simulink model "SWC_HALOUT_type_backup"  (R2021b)
settings: Solver=FixedStepDiscrete  StartTime=0.0  StopTime=10.0  FixedStep=0.001  RelTol=1e-3
undefined symbols (not defined in the file or in its folder): DIDLen_APPPedalZP, DIDLen_APSFunConfig, DIDLen_AutoLock, DIDLen_AutoWipHSpdEN, DIDLen_DKCKey, DIDLen_DRLDis, DIDLen_DynoMode, DIDLen_FMHTimer, DIDLen_LFLowPresThre, DIDLen_LFSensorID, DIDLen_LRLowPresThre, DIDLen_LRSensorID, DIDLen_NVMPedalZP, DIDLen_RFLowPresThre, DIDLen_RFSensorID, DIDLen_RRLowPresThre, DIDLen_RRSensorID, DIDLen_SensorMode, DIDLen_TireSize, DIDLen_TPMSLearnSta, DIDLen_TurnLampFLThreCurr, DIDLen_TurnLampFRThreCurr, DIDLen_TurnLampRLThreCurr, DIDLen_TurnLampRRThreCurr, DIDLen_USSConfig, DIDLen_WhlPres, DIDLen_WhlSensorBattSta, DIDLen_WhlTmp, DIDLen_WipRLSCmdCutFilter, DIDLen_WipRLSCmdHoldFilter, DIDLen_XWDMode, DIDNum_APPPedalZP, DIDNum_APSFunConfig, DIDNum_AutoLock, DIDNum_AutoWipHSpdEN, DIDNum_DKCKey, DIDNum_DRLDis, DIDNum_DynoMode, DIDNum_FMHTimer, DIDNum_LFLowPresThre, DIDNum_LFSensorID, DIDNum_LRLowPresThre, DIDNum_LRSensorID, DIDNum_NVMPedalZP, DIDNum_RFLowPresThre, DIDNum_RFSensorID, DIDNum_RRLowPresThre, DIDNum_RRSensorID, DIDNum_SensorMode, DIDNum_TireSize, DIDNum_TPMSLearnSta, DIDNum_TurnLampFLThreCurr, DIDNum_TurnLampFRThreCurr, DIDNum_TurnLampRLThreCurr, DIDNum_TurnLampRRThreCurr, DIDNum_USSConfig, DIDNum_WhlPres, DIDNum_WhlSensorBattSta, DIDNum_WhlTmp, DIDNum_WipRLSCmdCutFilter ... (+278)
libraries: FVT_lib x133, simulink x108, hdlsllib x6, hcu_lib x5, halout x1
(part 2 of 7)

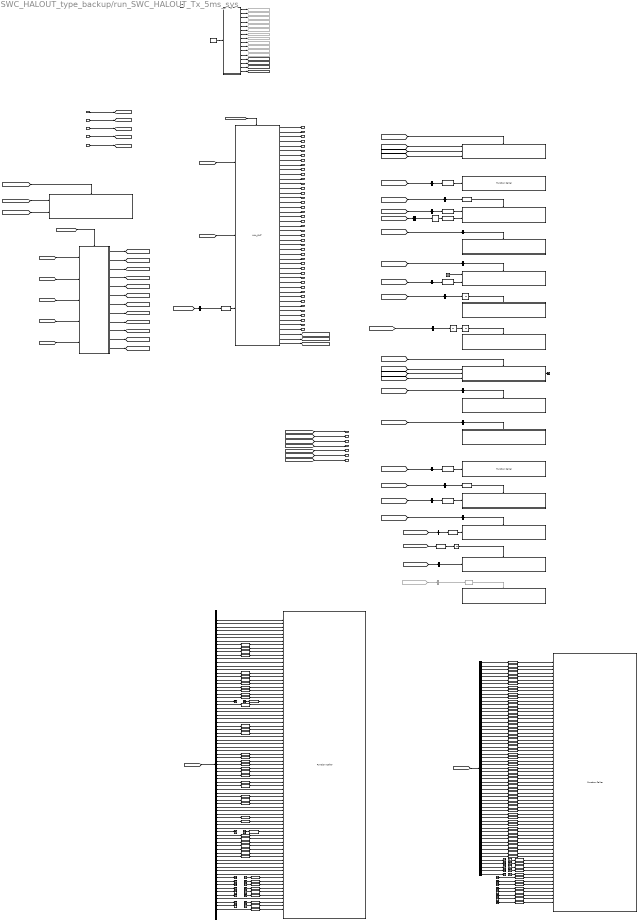
== system SWC_HALOUT_type_backup/run_SWC_HALOUT_Tx_5ms_sys ==
  R_BSCP_outputs_BSCP_outputs_read : Inport
  R_BOUTP_outputs_BOUTP_outputs_read : Inport  Port=2
  R_BHAL_SYS_outputs_BHAL_SYS_outputs_read : Inport  Port=3
  R_BHAL_DID_outputs_BHAL_DID_outputs_read : Inport  Port=4
  R_NVMReadCDD_u8Array1024_NVMReadData_read : Inport  Port=5
  function : TriggerPort  TriggerType=function-call  VariantControl=(inherit)  SampleTimeType=periodic  SampleTime=-1
  Bus Selector15 : BusSelector  OutputSignals=VHAL_AcoreReadyToSlp_flg
  Bus Selector3 : BusSelector  OutputSignals=VOUTP_PowerSta_enum,VOUTP_BrkPedalPos_pct,VOUTP_ActAPSPosn_pct,VOUTP_LFRawWhlSpeed_kph,VOUTP_RFRawWhlSpeed_kph,VOUTP_LRRawWhlSpeed_kph,VOUTP_RRRawWhlSpeed_kph,VOUTP_LFRawWhlSpeedV_flg,VOUTP_RFRawWhlSpeedV_flg,VOUTP_LRRawWhlSpeedV_flg,VOUTP_RRRawWhlSpeedV_flg,VOUTP_LFWhlRotDir_enum,VOUTP_RFWhlRotDir_enum,VOUTP_LRWhlRotDir_enum,VOUTP_RRWhlRotDir_enum,VOUTP_LFPulseCountV_flg,VOUTP_RFPulseCountV_flg,VOUTP_LRPulseCountV_flg,VOUTP_RRPulseCountV_flg,VOUTP_LFPulseCount_enum,VOUTP_RFPulseCount_enum,VOUTP_LRPulseCount_enum,VOUTP_RRPulseCount_enum,VOUTP_VehSpeed_kph,VOUTP_APSCtrlAvail_flg,VOUTP_ShifterHandleCmd_enum,VOUTP_DriIntend_enum,VOUTP_EPSAOIControl_enum,VOUTP_SASAngle_Deg,VOUTP_SASSpeed_degps,VOUTP_SASSpeedValid_flg,VOUTP_SASCAL_flg,VOUTP_SASV_flg,VOUTP_GRADE_Deg,VOUTP_YawRate_degps,VOUTP_LatAccel_Gps,VOUTP_LongAccel_Gps,VOUTP_MCPressure_bar,VOUTP_YawRateV_flg,VOUTP_LatAccelV_flg,VOUTP_LongAccelV_flg,VOUTP_MCPressureV_bar,VOUTP_BrkSwSta_flg,VOUTP_BrkSwV_flg,VOUTP_ESCStandstill_flg,VOUTP_ESCAPSSta_enum,VOUTP_EPBExtReleaseAvail_flg,VOUTP_EPBExtApplyAvail_flg,VOUTP_EPBErrSta_enum,VOUTP_EPBSta_enum,VOUTP_AllDoorSW_flg,VOUTP_HoodSW_flg,VOUTP_TailgateSW_flg,VOUTP_AVMparkingcancel_enum,VOUTP_AVMparkingexcute_enum,VOUTP_AVMParkingmode_enum,VOUTP_AVMErrSTA_flg,VOUTP_IVIStatus_flg,VOUTP_CAASSw_enum,VOUTP_IVIScreen_enum,VOUTP_VehSpeedTimeOut_flg,VOUTP_ABSActive_flg,VOUTP_TCSActive_flg,VOUTP_DriverSeatBeltCmd_flg,VOUTP_DrDoorSW_flg,VOUTP_PsDoorSW_flg,VOUTP_RLDoorSW_flg,VOUTP_RRDoorSW_flg,VOUTP_RFPressIndi_enum,VOUTP_LFPressIndi_enum,VOUTP_RRPressIndi_enum,VOUTP_LRPressIndi_enum,VOUTP_sigAmbAirT_C,VOUTP_FSOffSw_enum,VOUTP_FSOffSwTimeOut_flg,VOUTP_VehSpeed_kph,VOUTP_VehSpeed_kph,VOUTP_VehSpeed_kph,VOUTP_VehSpeed_kph,VOUTP_DrSeatSta_enum,VOUTP_VehSpeed_kph,VOUTP_VehSpeed_kph,VOUTP_IVIUserTakeOverAPSSta_flg
  Bus Selector4 : BusSelector  OutputSignals=VOUTP_BrkPedalPosTimeOut_flg,VOUTP_LFRawWhlSpeedTimeOut_flg,VOUTP_RFRawWhlSpeedTimeOut_flg,VOUTP_LRRawWhlSpeedTimeOut_flg,VOUTP_RRRawWhlSpeedTimeOut_flg,VOUTP_LFRawWhlSpeedVTimeOut_flg,VOUTP_RFRawWhlSpeedVTimeOut_flg,VOUTP_LRRawWhlSpeedVTimeOut_flg,VOUTP_RRRawWhlSpeedVTimeOut_flg,VOUTP_LFWhlRotDirTimeOut_flg,VOUTP_RFWhlRotDirTimeOut_flg,VOUTP_LRWhlRotDirTimeOut_flg,VOUTP_RRWhlRotDirTimeOut_flg,VOUTP_LFPulseCountVTimeOut_flg,VOUTP_RFPulseCountVTimeOut_flg,VOUTP_LRPulseCountVTimeOut_flg,VOUTP_RRPulseCountVTimeOut_flg,VOUTP_LFPulseCountTimeOut_flg,VOUTP_RFPulseCountTimeOut_flg,VOUTP_LRPulseCountTimeOut_flg,VOUTP_RRPulseCountTimeOut_flg,VOUTP_ShifterHandleCmdTimeOut_flg,VOUTP_DriIntendTimeOut_flg,VOUTP_EPSAOIControlTimeOut_flg,VOUTP_SASAngleTimeOut_flg,VOUTP_SASSpeedTimeOut_flg,VOUTP_SASSpeedValidTimeOut_flg,VOUTP_SASCALTimeOut_flg,VOUTP_SASVTimeOut_flg,VOUTP_GRADETimeOut_flg,VOUTP_YawRateTimeOut_flg,VOUTP_LatAccelTimeOut_flg,VOUTP_LongAccelTimeOut_flg,VOUTP_MCPressureTimeOut_flg,VOUTP_YawRateVTimeOut_flg,VOUTP_LatAccelVTimeOut_flg,VOUTP_LongAccelVTimeOut_flg,VOUTP_MCPressureVTimeOut_flg,VOUTP_BrkSwStaTimeOut_flg,VOUTP_BrkSwVTimeOut_flg,VOUTP_ESCStandstillTimeOut_flg,VOUTP_ESCAPSStaTimeOut_flg,VOUTP_EPBExtReleaseAvailTimeOut_flg,VOUTP_EPBExtApplyAvailTimeOut_flg,VOUTP_EPBErrStaTimeOut_flg,VOUTP_EPBStaTimeOut_flg,VOUTP_AVMparkingcancelTimeOut_flg,VOUTP_AVMparkingexcuteTimeOut_flg,VOUTP_AVMParkingmodeTimeOut_flg,VOUTP_AVMErrSTATimeOut_flg,VOUTP_IVIStatusTimeOut_flg,VOUTP_CAASSwTimeOut_flg,VOUTP_IVIScreenTimeOut_flg,VOUTP_ABSActiveTimeOut_flg,VOUTP_TCSActiveTimeOut_flg,VOUTP_DriverSeatBeltCmdTimeOut_flg,VOUTP_RFPressIndi_enum,VOUTP_LFPressIndi_enum,VOUTP_RRPressIndi_enum,VOUTP_LRPressIndi_enum,VOUTP_sigAmbAirT_C
  Bus Selector6 : BusSelector  OutputSignals=VHAL_TPMSSensorIDRegResults_raw8
  Bus Selector8 : BusSelector  Commented=on  OutputSignals=VOUTP_ResetPedalZeroPosStart_flg
  Bus Selector9 : BusSelector  OutputSignals=VHAL_DIDSetNVMPedalZP_raw8
  Constant5 : Constant  Value=FALSE
  DIDSet_Subsystem : Subsystem
  Data Type Conversion{,1..2,4..5,7..13,17..19,21..107,109..125} (119 alike) : DataTypeConversion  OutDataTypeStr=uint8
  Data Type Conversion108 : DataTypeConversion  OutDataTypeStr=boolean
  Data Type Conversion{14..16,20} (4 alike) : DataTypeConversion  OutDataTypeStr=int16
  Data Type Conversion3 : DataTypeConversion  OutDataTypeStr=uint32
  Data Type Conversion6 : DataTypeConversion  OutDataTypeStr=single
  Detect Increase1 : simulink/Logic and Bit Operations/Detect Increase  Commented=on  vinit=0.0  OutDataTypeStr=boolean
  From139 : From  Commented=on  GotoTag=BOUTP_outputs
  Goto100 : Goto  Commented=on  GotoTag=trig_Read_NVM_00
  Goto102 : Goto  Commented=on  GotoTag=trig_ReadIMUOffset_00
  Goto106 : Goto  Commented=on  GotoTag=trig_GetNMID
  Goto119 : Goto  Commented=on  GotoTag=trig_HAL_DKC_10_3
  Goto90 : Goto  Commented=on  GotoTag=trig_GetDID
  Goto91 : Goto  Commented=on  GotoTag=trig_WDG
  Goto92 : Goto  Commented=on  GotoTag=trig_HAL_DKC_10_2
  Goto93 : Goto  Commented=on  GotoTag=trig_HAL_CDD_10_1
  Goto96 : Goto  Commented=on  GotoTag=trig_OUTP_40
  Goto97 : Goto  Commented=on  GotoTag=trig_APP_30
  Goto98 : Goto  Commented=on  GotoTag=trig_INP_20
  Goto99 : Goto  Commented=on  GotoTag=trig_HAL_IN_10
  Ground{,1..8,10} (10 alike) : Ground
  Ground_{11..14,16..24,26} (14 alike) : Ground
  HALOUT_AFTER : Subsystem
  HAL_OUT : halout/HAL_OUT  SystemSampleTime=-1  VariantActivationTime=update diagram  Latency=0  AutoFrameSizeCalculation=off
  NOT : Logic  Operator=NOT  Inputs=1  AllPortsSameDT=off  OutDataTypeStr=boolean
  OUTP_AFTER : Subsystem
      settings: RTWSystemCode=Nonreusable function  RTWFcnNameOpts=Use subsystem name  RTWFileNameOpts=Use subsystem name
  R_DIDWriteCDD_CSOP_DIDSet_NVMPedalZP : Subsystem
  R_FDCCDD_Inner_CSOP_FDC_AppCallSleep : Subsystem
  R_HALOUTCDD_CSOP_AppNmStateReq : Subsystem
  R_HALOUTCDD_CSOP_ResetPedalZeroPosDone : Subsystem
  R_HALOUTCDD_CSOP_SetAcoreRebootCmdACK : Subsystem
  R_HALOUTCDD_CSOP_SetHazardIND : FunctionCaller  FunctionPrototype=R_HALOUTCDD_CSOP_SetHazardIND(u8_HazardIND)  InputArgumentSpecifications=uint8(1)
  R_HALOUTCDD_CSOP_SetSysPwrStat : FunctionCaller  FunctionPrototype=R_HALOUTCDD_CSOP_SetSysPwrStat(u8_SysPwrStat)  InputArgumentSpecifications=uint8(1)
  R_HALOUTCDD_CSOP_SleepRequest : Subsystem
  R_HALOUTCDD_CSOP_TPMSSensorIDRegSetResults : Subsystem
  R_HALOUT_APS_CSOP_ApsSetData : FunctionCaller  FunctionPrototype=R_HALOUT_APS_CSOP_ApsSetData(u8_SetPwrSta,f32_SetBrkPedalPos,f32_SetActAPSPosn,f32_SetLF_RawWhlSpeed,f32_SetRF_RawWhlSpeed,f32_SetLR_RawWhlSpeed,f32_SetRR_RawWhlSpeed,u8_SetLF_RawWhlSpeed_V,u8_SetRF_RawWhlSpeed_V,u8_SetLR_RawWhlSpeed_V,u8_SetRR_RawWhlSpeed_V,u8_SetLF_WhlRotDir,u8_SetRF_WhlRotDir,u8_SetLR_WhlRotDir,u8_SetRR_WhlRotDir,u8_SetLF_PulseCount_V,u8_SetRF_PulseCount_V,u8_SetLR_PulseCount_V,u8_SetRR_PulseCount_V,s16_SetLF_PulseCount,s16_SetRF_PulseCount,s16_SetLR_PulseCount,s16_SetRR_PulseCount,u8_SetAPS_Active,u8_SetAPS_CtrlAvail,u8_SetShifter_Handle_Cmd,u8_SetDriIntend,u8_SetEPS_AOI_Control,f32_SetSAS_Angle,f32_SetSAS_Speed,u8_SetSAS_Speed_Valid,u8_SetSAS_CAL,u8_SetSAS_OK,f32_SetGRADE,f32_SetYawRate,f32_SetLatAccel,f32_SetLongAccel,f32_SetMCPressure,u8_SetYawRate_V,u8_SetLatAccel_V,u8_SetLongAccel_V,u8_SetMCPressure_V,u8_SetBrkSw_Sta,u8_SetBrkSw_V,u8_SetESC_Standstill,u8_SetESC_APS_Sta,u8_SetEPBExtReleaseAvail,u8_SetEPBExtApplyAvail,u8_SetEPBErrSta,u8_SetEPBSta,u8_SetAllDoorSW,u8_SetHoodSW,u8_SetTailgate_SW,u8_SetAVM_parking_cancel,u8_SetAVM_parking_excute,u8_SetAVM_Parking_mode,u8_SetAVM_Err_STA,u8_SetIVI_Status,u8_SetCAAS_Sw,u8_SetIVI_Screen,u8_SetCAAS_CtrlAvail,u8_SetABS_Active,u8_SetTCS_Active,u8_SetDriverSeatBeltCmd,u8_SetDrDoorSW,u8_SetPsDoorSW,u8_SetRLDoorSW,u8_SetRRDoorSW,u8_SetRFPressIndi,u8_SetLFPressIndi,u8_SetRRPressIndi,u8_SetLRPressIndi,f32_SetsigAmbAirT,f32_SetVehActSpd,u8_SetCAAS_Active,u8_SetAPS_PwrReqAvail_sta,u8_SetDKC_PDkeyAreaRAPS_Sta,u8_SetDKC_ParkingMode_Cmd,u8_SetP_UID_LowPower,u8_SetDr_SeatSta,u8_SetVCU_RAPSErrLv2_flg,u8_SetVCU_RAPSErrLv3_flg,u8_SetIVI_UserTakeOver_APS_Sta)  InputArgumentSpecifications=uint8(1), single(1), single(1), single(1), single(1), single(1), single(1), uint8(1), uint8(1), uint8(1), uint8(1), uint8(1), uint8(1), uint8(1), uint8(1), uint8(1), uint8(1), uint8(1), uint8(1), int16(1), int16(1), int16(1), int16(1), uint8(1), uint8(1), uint8(1), uint8(1), uint8(1), single(1), single(1), uint8(1), uint8(1), uint8(1), single(1), single(1), single(1), single(1), single(1), uint8(1), uint8(1), uint8(1), uint8(1), uint8(1), uint8(1), uint8(1), uint8(1), uint8(1), uint8(1), uint8(1), uint8(1), uint8(1), uint8(1), uint8(1), uint8(1), uint8(1), uint8(1), uint8(1), uint8(1), uint8(1), uint8(1), uint8(1), uint8(1), uint8(1), uint8(1), uint8(1), uint8(1), uint8(1), uint8(1), uint8(1), uint8(1), uint8(1), uint8(1), single(1), single(1), uint8(1), uint8(1), uint8(1), uint8(1), uint8(1), uint8(1), uint8(1), uint8(1), uint8(1)
  R_HALOUT_APS_CSOP_ApsSetTimeout : FunctionCaller  FunctionPrototype=R_HALOUT_APS_CSOP_ApsSetTimeout(u8_SetBrkPedalPosTO,u8_SetLF_RawWhlSpeedTO,u8_SetRF_RawWhlSpeedTO,u8_SetLR_RawWhlSpeedTO,u8_SetRR_RawWhlSpeedTO,u8_SetLF_RawWhlSpeed_VTO,u8_SetRF_RawWhlSpeed_VTO,u8_SetLR_RawWhlSpeed_VTO,u8_SetRR_RawWhlSpeed_VTO,u8_SetLF_WhlRotDirTO,u8_SetRF_WhlRotDirTO,u8_SetLR_WhlRotDirTO,u8_SetRR_WhlRotDirTO,u8_SetLF_PulseCount_VTO,u8_SetRF_PulseCount_VTO,u8_SetLR_PulseCount_VTO,u8_SetRR_PulseCount_VTO,u8_SetLF_PulseCountTO,u8_SetRF_PulseCountTO,u8_SetLR_PulseCountTO,u8_SetRR_PulseCountTO,u8_SetShifter_Handle_CmdTO,u8_SetDriIntendTO,u8_SetEPS_AOI_ControlTO,u8_SetSAS_AngleTO,u8_SetSAS_SpeedTO,u8_SetSAS_Speed_ValidTO,u8_SetSAS_CALTO,u8_SetSAS_OKTO,u8_SetGRADETO,u8_SetYawRateTO,u8_SetLatAccelTO,u8_SetLongAccelTO,u8_SetMCPressureTO,u8_SetYawRate_VTO,u8_SetLatAccel_VTO,u8_SetLongAccel_VTO,u8_SetMCPressure_VTO,u8_SetBrkSw_StaTO,u8_SetBrkSw_VTO,u8_SetESC_StandstillTO,u8_SetESC_APS_StaTO,u8_SetEPBExtReleaseAvailTO,u8_SetEPBExtApplyAvailTO,u8_SetEPBErrStaTO,u8_SetEPBStaTO,u8_SetAVM_parking_cancelTO,u8_SetAVM_parking_excuteTO,u8_SetAVM_Parking_modeTO,u8_SetAVM_Err_STATO,u8_SetIVI_StatusTO,u8_SetCAAS_SwTO,u8_SetIVI_ScreenTO,u8_SetABS_ActiveTO,u8_SetTCS_ActiveTO,u8_SetDriverSeatBeltCmdTO,u8_SetRFPressIndiTO,u8_SetLFPressIndiTO,u8_SetRRPressIndiTO,u8_SetLRPressIndiTO,u8_SetsigAmbAirTTO,u8_SetAPS_PwrReqAvail_staTO,u8_SetDKC_PDkeyAreaRAPS_StaTO,u8_SetDKC_ParkingMode_CmdTO,u8_SetP_UID_LowPowerTO,u8_SetDr_SeatStaTO,u8_SetVCU_RAPSErrLv2_flgTO,u8_SetVCU_RAPSErrLv3_flgTO,u8_SetIVI_UserTakeOver_APS_StaTO)  InputArgumentSpecifications=uint8(1), uint8(1), uint8(1), uint8(1), uint8(1), uint8(1), uint8(1), uint8(1), uint8(1), uint8(1), uint8(1), uint8(1), uint8(1), uint8(1), uint8(1), uint8(1), uint8(1), uint8(1), uint8(1), uint8(1), uint8(1), uint8(1), uint8(1), uint8(1), uint8(1), uint8(1), uint8(1), uint8(1), uint8(1), uint8(1), uint8(1), uint8(1), uint8(1), uint8(1), uint8(1), uint8(1), uint8(1), uint8(1), uint8(1), uint8(1), uint8(1), uint8(1), uint8(1), uint8(1), uint8(1), uint8(1), uint8(1), uint8(1), uint8(1), uint8(1), uint8(1), uint8(1), uint8(1), uint8(1), uint8(1), uint8(1), uint8(1), uint8(1), uint8(1), uint8(1), uint8(1), uint8(1), uint8(1), uint8(1), uint8(1), uint8(1), uint8(1), uint8(1), uint8(1)
  R_IOExpOUT_CDD_CSOP_IOExpSetVal : Subsystem
  R_NVMWriteCDD_Inner_NVM_WriteOperation : Subsystem
  R_UDSCDD_CSOP_DdmRestartOperationCycle : Subsystem
  R_UDSCDD_CSOP_SetDTCStatus : Subsystem
  R_WDGCDD_CSOP_Call_WDG_AppEnd : Subsystem
  Terminator{,1..8,10..15} (15 alike) : Terminator
  Terminator_16 : Terminator
  Unit Delay{,1..2,4} (4 alike) : UnitDelay  SampleTime=-1  HasFrameUpgradeWarning=on
  bus_selector : BusSelector  OutputSignals=VOUTP_SysPowerMode_enum
  bus_selector1 : BusSelector  OutputSignals=VOUTP_NetworkReq_flg
  bus_selector10 : BusSelector  OutputSignals=VOUTP_AcoreRebootCmdACK_flg
  bus_selector11 : BusSelector  OutputSignals=VOUTP_HazardIND_flg
  bus_selector12 : BusSelector  OutputSignals=VOUTP_IVIRST_flg
  bus_selector13 : BusSelector  OutputSignals=VOUTP_IVIRST_flg
  bus_selector14 : BusSelector  OutputSignals=VOUTP_TPMSSensorIDRegStart_flg
  bus_selector2 : BusSelector  OutputSignals=VOUTP_NetworkReq_flg
  bus_selector3 : BusSelector  OutputSignals=VOUTP_NetworkReq_flg
  bus_selector4 : BusSelector  OutputSignals=VOUTP_NvWriteReqRisingEdge_flg
  bus_selector5 : BusSelector  OutputSignals=VOUTP_FdcSlpTime_sec
  bus_selector6 : BusSelector  OutputSignals=VOUTP_FdcSlpReqRisingEdge_flg
  bus_selector7 : BusSelector  OutputSignals=VOUTP_FdcSlpReqRisingEdge_flg
  bus_selector8 : BusSelector  OutputSignals=VOUTP_FdcSlpReqRisingEdge_flg
  bus_selector9 : BusSelector  OutputSignals=VOUTP_EnterNewOperCyc_flg
  detect_change : simulink/Logic and Bit Operations/Detect Change  vinit=0  OutDataTypeStr=boolean
  detect_change1 : simulink/Logic and Bit Operations/Detect Change  vinit=0  OutDataTypeStr=boolean
  hcu_main_sched : Stateflow chart  TreatAsAtomicUnit=on
  P_CAN1_FD1_BCM1_CAN1_SG_FD1_BCM1_write : Outport
  P_CAN1_FD1_VCU1_CAN1_SG_FD1_VCU1_write : Outport  Port=2
  P_CAN1_FD1_VMC1_CAN1_SG_FD1_VMC1_write : Outport  Port=3
  P_CAN2_FD2_CE100_0_CAN2_SG_FD2_CE100_0_write : Outport  Port=4
  P_CAN2_FD2_CE200_1_CAN2_SG_FD2_CE200_1_write : Outport  Port=5
  P_CAN2_GW2_CE100_0_CAN2_SG_GW2_CE100_0_write : Outport  Port=6
  P_CAN2_GW2_CE200_0_CAN2_SG_GW2_CE200_0_write : Outport  Port=7
  P_CAN3_FD3_BCM1_CAN3_SG_FD3_BCM1_write : Outport  Port=8
  P_CAN3_FD3_THCM2_CAN3_SG_FD3_THCM2_write : Outport  Port=9
  P_CAN3_FD3_V2L1_CAN3_SG_FD3_V2L1_write : Outport  Port=10
  P_CAN4_FD4_CE100_1_CAN4_SG_FD4_CE100_1_write : Outport  Port=11
  P_CAN4_FD4_CE200_0_CAN4_SG_FD4_CE200_0_write : Outport  Port=12
  P_CAN4_GW4_CE100_0_CAN4_SG_GW4_CE100_0_write : Outport  Port=13
  P_CAN5_FD5_CE100_0_CAN5_SG_FD5_CE100_0_write : Outport  Port=14
  P_CAN5_FD5_Debug1_CAN5_SG_FD5_Debug1_write : Outport  Port=15
  P_CAN5_FD5_Debug2_CAN5_SG_FD5_Debug2_write : Outport  Port=16
  P_CAN6_FD6_BCM1_CAN6_SG_FD6_BCM1_write : Outport  Port=17
  P_CAN6_FD6_VCU1_CAN6_SG_FD6_VCU1_write : Outport  Port=18
  P_CAN6_FD6_VMC1_CAN6_SG_FD6_VMC1_write : Outport  Port=19
  P_CAN6_GW6_CE100_0_CAN6_SG_GW6_CE100_0_write : Outport  Port=20
  IRV_ms10_CAN1_SG_FD1_APS3_write : Outport  Port=21  OutDataTypeStr=Bus: DT_CAN1_SG_FD1_APS3  PortDimensions=1  BusOutputAsStruct=on
  IRV_ms10_CAN1_SG_FD1_VCU2_write : Outport  Port=22  OutDataTypeStr=Bus: DT_CAN1_SG_FD1_VCU2  PortDimensions=1  BusOutputAsStruct=on
  IRV_ms10_CAN1_SG_FD1_VCU3_write : Outport  Port=23  OutDataTypeStr=Bus: DT_CAN1_SG_FD1_VCU3  PortDimensions=1  BusOutputAsStruct=on
  IRV_ms10_CAN1_SG_VMC_FCM1_write : Outport  Port=24  OutDataTypeStr=Bus: DT_CAN1_SG_VMC_FCM1  PortDimensions=1  BusOutputAsStruct=on
  IRV_ms10_CAN3_SG_FD3_VCU0_write : Outport  Port=25  OutDataTypeStr=Bus: DT_CAN3_SG_FD3_VCU0  PortDimensions=1  BusOutputAsStruct=on
  IRV_ms10_CAN3_SG_FD3_VCU2_write : Outport  Port=26  OutDataTypeStr=Bus: DT_CAN3_SG_FD3_VCU2  PortDimensions=1  BusOutputAsStruct=on
  IRV_ms10_CAN3_SG_FD3_VCU2_toNIDEC_write : Outport  Port=27  OutDataTypeStr=Bus: DT_CAN3_SG_FD3_VCU2_toNIDEC  PortDimensions=1  BusOutputAsStruct=on
  IRV_ms10_CAN3_SG_FD3_VCU5_write : Outport  Port=28  OutDataTypeStr=Bus: DT_CAN3_SG_FD3_VCU5  PortDimensions=1  BusOutputAsStruct=on
  IRV_ms10_CAN3_SG_GW_ESC1_toNIDEC_write : Outport  Port=29  OutDataTypeStr=Bus: DT_CAN3_SG_GW_ESC1_toNIDEC  PortDimensions=1  BusOutputAsStruct=on
  IRV_ms10_CAN5_SG_FD5_Debug3_write : Outport  Port=30  OutDataTypeStr=Bus: DT_CAN5_SG_FD5_Debug3  PortDimensions=1  BusOutputAsStruct=on
  IRV_ms10_CAN6_SG_FD6_APS3_write : Outport  Port=31  OutDataTypeStr=Bus: DT_CAN6_SG_FD6_APS3  PortDimensions=1  BusOutputAsStruct=on
  IRV_ms10_CAN6_SG_FD6_VCU2_write : Outport  Port=32  OutDataTypeStr=Bus: DT_CAN6_SG_FD6_VCU2  PortDimensions=1  BusOutputAsStruct=on
  IRV_ms100_CAN1_SG_FD1_THCM1_write : Outport  Port=33  OutDataTypeStr=Bus: DT_CAN1_SG_FD1_THCM1  PortDimensions=1  BusOutputAsStruct=on
  IRV_ms100_CAN3_SG_FD3_THCM1_write : Outport  Port=34  OutDataTypeStr=Bus: DT_CAN3_SG_FD3_THCM1  PortDimensions=1  BusOutputAsStruct=on
  IRV_ms1000_CAN3_SG_GW_IVI6_toNIDEC_write : Outport  Port=35  OutDataTypeStr=Bus: DT_CAN3_SG_GW_IVI6_toNIDEC  PortDimensions=1  BusOutputAsStruct=on
  IRV_ms20_CAN1_SG_FD1_APS2_write : Outport  Port=36  OutDataTypeStr=Bus: DT_CAN1_SG_FD1_APS2  PortDimensions=1  BusOutputAsStruct=on
  IRV_ms20_CAN2_SG_FD2_C20_0_write : Outport  Port=37  OutDataTypeStr=Bus: DT_CAN2_SG_FD2_C20_0  PortDimensions=1  BusOutputAsStruct=on
  IRV_ms500_CAN1_SG_FD1_VMC2_write : Outport  Port=38  OutDataTypeStr=Bus: DT_CAN1_SG_FD1_VMC2  PortDimensions=1  BusOutputAsStruct=on
  IRV_ms5000_CAN2_SG_FD2_Version_write : Outport  Port=39  OutDataTypeStr=Bus: DT_CAN2_SG_FD2_Version  PortDimensions=1  BusOutputAsStruct=on
  IRV_E2E_CAN3_SG_FD3_VCU1_write : Outport  Port=40  OutDataTypeStr=Bus: DT_CAN3_SG_FD3_VCU1  PortDimensions=1  BusOutputAsStruct=on
  IRV_E2E_CAN3_SG_FD3_VCU1_toNIDEC_write : Outport  Port=41  OutDataTypeStr=Bus: DT_CAN3_SG_FD3_VCU1_toNIDEC  PortDimensions=1  BusOutputAsStruct=on
  IRV_E2E_CAN4_SG_FD4_CE100_0_write : Outport  Port=42  OutDataTypeStr=Bus: DT_CAN4_SG_FD4_CE100_0  PortDimensions=1  BusOutputAsStruct=on
  IRV_f32_ApsOutVehSpdSig_write : Outport  Port=43  OutDataTypeStr=single  PortDimensions=1
  IRV_u8Array1024_NvmWriteArray_write : Outport  Port=44  OutDataTypeStr=uint8  PortDimensions=1024
  IRV_u8_ApsOutGearPosnSig_write : Outport  Port=45  OutDataTypeStr=uint8  PortDimensions=1
  IRV_u8_ApsOutSendChrgPlugSta_write : Outport  Port=46  OutDataTypeStr=uint8  PortDimensions=1
  IRV_u8_ApsOutSetFrSensorOnCmd_write : Outport  Port=47  OutDataTypeStr=uint8  PortDimensions=1
  IRV_u8_ApsOutSetFrSensorSwTOCmd_write : Outport  Port=48  OutDataTypeStr=uint8  PortDimensions=1
  IRV_u8_ApsOutSetVehSpdTOCmd_write : Outport  Port=49  OutDataTypeStr=uint8  PortDimensions=1
  IRV_ms100_CAN2_SG_GW2_CE100_1_write : Outport  Port=50  OutDataTypeStr=Bus: DT_CAN2_SG_GW2_CE100_1  PortDimensions=1  BusOutputAsStruct=on
  IRV_ms100_CAN5_SG_GW5_CE100_0_write : Outport  Port=51  OutDataTypeStr=Bus: DT_CAN5_SG_GW5_CE100_0  PortDimensions=1  BusOutputAsStruct=on
  wires:
  [f32_ApsOutVehSpdSig] -> IRV_f32_ApsOutVehSpdSig_write/1
  [u8Array1024_NvmWriteArray] -> IRV_u8Array1024_NvmWriteArray_write/1
  [u8_ApsOutGearPosnSig] -> IRV_u8_ApsOutGearPosnSig_write/1
  [u8_ApsOutSendChrgPlugSta] -> IRV_u8_ApsOutSendChrgPlugSta_write/1
  [u8_ApsOutSetFrSensorOnCmd] -> IRV_u8_ApsOutSetFrSensorOnCmd_write/1
  [u8_ApsOutSetFrSensorSwTOCmd] -> IRV_u8_ApsOutSetFrSensorSwTOCmd_write/1
  [u8_ApsOutSetVehSpdTOCmd] -> IRV_u8_ApsOutSetVehSpdTOCmd_write/1
  Data Type Conversion/1 -> R_HALOUTCDD_CSOP_SetSysPwrStat/1
  bus_selector/1 -> Data Type Conversion/1  "<VOUTP_SysPowerMode_enum>"
  [BOUTP_outputs] -> bus_selector/1
  Data Type Conversion1/1 -> R_HALOUTCDD_CSOP_AppNmStateReq/1(WakeReq)
  bus_selector1/1 -> Data Type Conversion1/1  "<VOUTP_NetworkReq_flg>"
  [BOUTP_outputs] -> bus_selector1/1
  Data Type Conversion2/1 -> R_HALOUTCDD_CSOP_AppNmStateReq/2(SleepReq)
  NOT/1 -> Data Type Conversion2/1
  bus_selector2/1 -> NOT/1  "<VOUTP_NetworkReq_flg>"
  [BOUTP_outputs] -> bus_selector2/1
  detect_change/1 -> R_HALOUTCDD_CSOP_AppNmStateReq/Enable
  bus_selector3/1 -> detect_change/1  "<VOUTP_NetworkReq_flg>"
  [BOUTP_outputs] -> bus_selector3/1
  bus_selector4/1 -> R_NVMWriteCDD_Inner_NVM_WriteOperation/Enable  "<VOUTP_NvWriteReqRisingEdge_flg>"
  [BOUTP_outputs] -> bus_selector4/1
  Data Type Conversion3/1 -> R_HALOUTCDD_CSOP_SleepRequest/2(WakeUpTime)
  bus_selector5/1 -> Data Type Conversion3/1  "<VOUTP_FdcSlpTime_sec>"
  [BOUTP_outputs] -> bus_selector5/1
  bus_selector6/1 -> R_HALOUTCDD_CSOP_SleepRequest/Enable  "<VOUTP_FdcSlpReqRisingEdge_flg>"
  [BOUTP_outputs] -> bus_selector6/1
  Unit Delay/1 -> R_WDGCDD_CSOP_Call_WDG_AppEnd/Enable
  bus_selector7/1 -> Unit Delay/1  "<VOUTP_FdcSlpReqRisingEdge_flg>"
  [BOUTP_outputs] -> bus_selector7/1
  Unit Delay1/1 -> R_FDCCDD_Inner_CSOP_FDC_AppCallSleep/Enable
  Unit Delay2/1 -> Unit Delay1/1
  bus_selector8/1 -> Unit Delay2/1  "<VOUTP_FdcSlpReqRisingEdge_flg>"
  [BOUTP_outputs] -> bus_selector8/1
  [Header_Array] -> R_UDSCDD_CSOP_SetDTCStatus/1(Header_Array)
  [DTC_Array] -> R_UDSCDD_CSOP_SetDTCStatus/2(DTC_Array)
  [DTC_Trigger] -> R_UDSCDD_CSOP_SetDTCStatus/Enable
  bus_selector9/1 -> R_UDSCDD_CSOP_DdmRestartOperationCycle/Enable  "<VOUTP_EnterNewOperCyc_flg>"
  [BOUTP_outputs] -> bus_selector9/1
  bus_selector10/1 -> R_HALOUTCDD_CSOP_SetAcoreRebootCmdACK/Enable  "<VOUTP_AcoreRebootCmdACK_flg>"
  [BOUTP_outputs] -> bus_selector10/1
  Data Type Conversion4/1 -> R_HALOUTCDD_CSOP_SetHazardIND/1
  bus_selector11/1 -> Data Type Conversion4/1  "<VOUTP_HazardIND_flg>"
  [BOUTP_outputs] -> bus_selector11/1
  Data Type Conversion5/1 -> R_IOExpOUT_CDD_CSOP_IOExpSetVal/1(In1)
  bus_selector12/1 -> Data Type Conversion5/1  "<VOUTP_IVIRST_flg>"
  [BOUTP_outputs] -> bus_selector12/1
  detect_change1/1 -> R_IOExpOUT_CDD_CSOP_IOExpSetVal/Enable
  bus_selector13/1 -> detect_change1/1  "<VOUTP_IVIRST_flg>"
  [BOUTP_outputs] -> bus_selector13/1
  bus_selector14/1 -> R_HALOUTCDD_CSOP_TPMSSensorIDRegSetResults/Enable  "<VOUTP_TPMSSensorIDRegStart_flg>"
  [BOUTP_outputs] -> bus_selector14/1
  [E2E_CAN3_VCU1_Trigger] -> HALOUT_AFTER/1(E2E_CAN3_VCU1_Trigger)
  [E2E_CAN3_VCU1_toNIDEC_Trigger] -> HALOUT_AFTER/2(E2E_CAN3_VCU1_Trigger_toNIDEC)
  [E2E_CAN4_VCU1_Trigger] -> HALOUT_AFTER/3(E2E_CAN4_VCU1_Trigger)
  [trig_HAL_OUTAFTER_50_1] -> HALOUT_AFTER/Trigger
  [BOUTP_DIDSetData_outputs] -> DIDSet_Subsystem/1(BOUTP_DIDSetData_outputs)
  [BHAL_DID_outputs] -> DIDSet_Subsystem/2(BHAL_DID_outputs)
  [trig_SetDID] -> DIDSet_Subsystem/Trigger
  [BOUTP_outputs] -> HAL_OUT/1
  [trig_HAL_OUT_50] -> HAL_OUT/Trigger
  Bus Selector15/1 -> Data Type Conversion125/1  "<VHAL_AcoreReadyToSlp_flg>"
  Data Type Conversion125/1 -> HAL_OUT/3
  [BSCP_outputs] -> HAL_OUT/2
  [BHAL_SYS_outputs] -> Bus Selector15/1
  HAL_OUT/1 -> P_CAN1_FD1_BCM1_CAN1_SG_FD1_BCM1_write/1
  HAL_OUT/2 -> P_CAN1_FD1_VCU1_CAN1_SG_FD1_VCU1_write/1
  HAL_OUT/3 -> P_CAN1_FD1_VMC1_CAN1_SG_FD1_VMC1_write/1
  HAL_OUT/4 -> P_CAN2_FD2_CE100_0_CAN2_SG_FD2_CE100_0_write/1
  HAL_OUT/5 -> P_CAN2_FD2_CE200_1_CAN2_SG_FD2_CE200_1_write/1
  HAL_OUT/6 -> P_CAN2_GW2_CE100_0_CAN2_SG_GW2_CE100_0_write/1
  HAL_OUT/7 -> P_CAN2_GW2_CE200_0_CAN2_SG_GW2_CE200_0_write/1
  HAL_OUT/8 -> P_CAN3_FD3_BCM1_CAN3_SG_FD3_BCM1_write/1
  HAL_OUT/9 -> P_CAN3_FD3_THCM2_CAN3_SG_FD3_THCM2_write/1
  HAL_OUT/10 -> P_CAN3_FD3_V2L1_CAN3_SG_FD3_V2L1_write/1
  HAL_OUT/11 -> P_CAN4_FD4_CE100_1_CAN4_SG_FD4_CE100_1_write/1
  HAL_OUT/12 -> P_CAN4_FD4_CE200_0_CAN4_SG_FD4_CE200_0_write/1
  HAL_OUT/13 -> P_CAN4_GW4_CE100_0_CAN4_SG_GW4_CE100_0_write/1
  HAL_OUT/14 -> P_CAN5_FD5_CE100_0_CAN5_SG_FD5_CE100_0_write/1
  HAL_OUT/15 -> P_CAN5_FD5_Debug1_CAN5_SG_FD5_Debug1_write/1
  HAL_OUT/16 -> P_CAN5_FD5_Debug2_CAN5_SG_FD5_Debug2_write/1
  HAL_OUT/17 -> P_CAN6_FD6_BCM1_CAN6_SG_FD6_BCM1_write/1
  HAL_OUT/18 -> P_CAN6_FD6_VCU1_CAN6_SG_FD6_VCU1_write/1
  HAL_OUT/19 -> P_CAN6_FD6_VMC1_CAN6_SG_FD6_VMC1_write/1
  HAL_OUT/20 -> P_CAN6_GW6_CE100_0_CAN6_SG_GW6_CE100_0_write/1
  HAL_OUT/21 -> IRV_ms10_CAN1_SG_FD1_APS3_write/1
  HAL_OUT/22 -> IRV_ms10_CAN1_SG_FD1_VCU2_write/1
  HAL_OUT/23 -> IRV_ms10_CAN1_SG_FD1_VCU3_write/1
  HAL_OUT/24 -> IRV_ms10_CAN1_SG_VMC_FCM1_write/1
  HAL_OUT/25 -> IRV_ms10_CAN3_SG_FD3_VCU0_write/1
  HAL_OUT/26 -> IRV_ms10_CAN3_SG_FD3_VCU2_write/1
  HAL_OUT/27 -> IRV_ms10_CAN3_SG_FD3_VCU2_toNIDEC_write/1
  HAL_OUT/28 -> IRV_ms10_CAN3_SG_FD3_VCU5_write/1
  HAL_OUT/29 -> IRV_ms10_CAN3_SG_GW_ESC1_toNIDEC_write/1
  HAL_OUT/30 -> IRV_ms10_CAN5_SG_FD5_Debug3_write/1
  HAL_OUT/31 -> IRV_ms10_CAN6_SG_FD6_APS3_write/1
  HAL_OUT/32 -> IRV_ms10_CAN6_SG_FD6_VCU2_write/1
  HAL_OUT/33 -> IRV_ms100_CAN1_SG_FD1_THCM1_write/1
  OUTP_AFTER/5(ApsOut_SetVehSpdTOCmd) -> [u8_ApsOutSetVehSpdTOCmd]
  OUTP_AFTER/2(ApsOut_SendChrgPlugStaSig) -> [u8_ApsOutSendChrgPlugSta]
  [u8Array1024_NvmReadArray] -> OUTP_AFTER/4(VHAL_NvmReadArray_raw)
  OUTP_AFTER/4(ApsOut_SetFrSensorSwTOCmd) -> [u8_ApsOutSetFrSensorSwTOCmd]
  OUTP_AFTER/7(HAL_NvmWriteData_raw) -> [u8Array1024_NvmWriteArray]
  OUTP_AFTER/8(DTC_Trigger) -> [DTC_Trigger]
  OUTP_AFTER/6(ApsOut_VehSpdSig) -> [f32_ApsOutVehSpdSig]
  OUTP_AFTER/11(BOUTP_DIDSetData_outputs) -> [BOUTP_DIDSetData_outputs]
  [trig_OUTP_AFTER_40_1] -> OUTP_AFTER/Trigger
  [BHAL_SYS_outputs] -> OUTP_AFTER/2(BHAL_SYSTPMS_outputs)
  OUTP_AFTER/3(ApsOut_SetFrSensorOnCmd) -> [u8_ApsOutSetFrSensorOnCmd]
  OUTP_AFTER/10(DTC_Array) -> [DTC_Array]
  [BHAL_DID_outputs] -> OUTP_AFTER/5(BHAL_DIDGetData_raw)
  [BHAL_SYS_outputs] -> OUTP_AFTER/3(BHAL_SYS_outputs)
  [BOUTP_outputs] -> OUTP_AFTER/1(BOUTP_outputs)
  OUTP_AFTER/9(Header_Array) -> [Header_Array]
  OUTP_AFTER/1(ApsOut_GearPosnSig) -> [u8_ApsOutGearPosnSig]
  R_BOUTP_outputs_BOUTP_outputs_read/1 -> [BOUTP_outputs]
  R_NVMReadCDD_u8Array1024_NVMReadData_read/1 -> [u8Array1024_NvmReadArray]
  R_BHAL_SYS_outputs_BHAL_SYS_outputs_read/1 -> [BHAL_SYS_outputs]
  R_BHAL_DID_outputs_BHAL_DID_outputs_read/1 -> [BHAL_DID_outputs]
  R_BSCP_outputs_BSCP_outputs_read/1 -> [BSCP_outputs]
  hcu_main_sched/2(trig_ReadIMUOffset_00()) -> Goto102/1
  hcu_main_sched/12(trig_OUTP_40()) -> Goto96/1
  hcu_main_sched/15(trig_HAL_OUT_50()) -> [trig_HAL_OUT_50]
  hcu_main_sched/9(trig_HAL_DKC_10_3()) -> Goto119/1
  hcu_main_sched/16(trig_HAL_OUTAFTER_50_1()) -> [trig_HAL_OUTAFTER_50_1]
  hcu_main_sched/1(trig_Read_NVM_00()) -> Goto100/1
  hcu_main_sched/6(trig_HAL_IN_10()) -> Goto99/1
  hcu_main_sched/10(trig_INP_20()) -> Goto98/1
  hcu_main_sched/11(trig_APP_30()) -> Goto97/1
  hcu_main_sched/14(trig_SetDID()) -> [trig_SetDID]
  hcu_main_sched/8(trig_HAL_DKC_10_2()) -> Goto92/1
  hcu_main_sched/4(trig_GetNMID()) -> Goto106/1
  Constant5/1 -> hcu_main_sched/1(VHAL_FusionSchedReq_flg)
  hcu_main_sched/5(trig_GetDID()) -> Goto90/1
  hcu_main_sched/3(trig_WDG()) -> Goto91/1
  hcu_main_sched/13(trig_OUTP_AFTER_40_1()) -> [trig_OUTP_AFTER_40_1]
  hcu_main_sched/7(trig_HAL_CDD_10_1()) -> Goto93/1
  Bus Selector3/17 -> Data Type Conversion11/1  "<VOUTP_RFPulseCountV_flg>"
  Data Type Conversion16/1 -> R_HALOUT_APS_CSOP_ApsSetData/23
  Bus Selector3/47 -> Data Type Conversion31/1  "<VOUTP_EPBExtReleaseAvail_flg>"
  Bus Selector3/80 -> R_HALOUT_APS_CSOP_ApsSetData/80  "<VOUTP_DrSeatSta_enum>"
  Bus Selector3/42 -> Data Type Conversion27/1  "<VOUTP_MCPressureV_bar>"
  Data Type Conversion30/1 -> R_HALOUT_APS_CSOP_ApsSetData/45
  Data Type Conversion119/1 -> R_HALOUT_APS_CSOP_ApsSetData/77
  Data Type Conversion15/1 -> R_HALOUT_APS_CSOP_ApsSetData/22
  Bus Selector3/4 -> R_HALOUT_APS_CSOP_ApsSetData/4  "<VOUTP_LFRawWhlSpeed_kph>"
  Bus Selector3/10 -> Data Type Conversion9/1  "<VOUTP_LRRawWhlSpeedV_flg>"
  Data Type Conversion100/1 -> R_HALOUT_APS_CSOP_ApsSetData/66
  Ground_12/1 -> Data Type Conversion119/1
  Bus Selector3/23 -> Data Type Conversion16/1  "<VOUTP_RRPulseCount_enum>"
  Bus Selector3/31 -> Data Type Conversion21/1  "<VOUTP_SASSpeedValid_flg>"
  Bus Selector3/78 -> Terminator12/1  "<VOUTP_VehSpeed_kph>"
  Bus Selector3/29 -> R_HALOUT_APS_CSOP_ApsSetData/29  "<VOUTP_SASAngle_Deg>"
  Bus Selector3/75 -> Terminator6/1  "<VOUTP_FSOffSwTimeOut_flg>"
  Bus Selector3/38 -> R_HALOUT_APS_CSOP_ApsSetData/38  "<VOUTP_MCPressure_bar>"
  Bus Selector3/25 -> Data Type Conversion18/1  "<VOUTP_APSCtrlAvail_flg>"
  Bus Selector3/79 -> Terminator11/1  "<VOUTP_VehSpeed_kph>"
  Ground/1 -> Data Type Conversion6/1
  Data Type Conversion117/1 -> R_HALOUT_APS_CSOP_ApsSetData/83
  Bus Selector3/74 -> Terminator/1  "<VOUTP_FSOffSw_enum>"
  Bus Selector3/57 -> Data Type Conversion36/1  "<VOUTP_AVMErrSTA_flg>"
  Bus Selector3/35 -> R_HALOUT_APS_CSOP_ApsSetData/35  "<VOUTP_YawRate_degps>"
  Data Type Conversion20/1 -> R_HALOUT_APS_CSOP_ApsSetData/20
  Bus Selector3/76 -> Terminator15/1  "<VOUTP_VehSpeed_kph>"
  Data Type Conversion21/1 -> R_HALOUT_APS_CSOP_ApsSetData/31
  Bus Selector3/73 -> R_HALOUT_APS_CSOP_ApsSetData/73  "<VOUTP_sigAmbAirT_C>"
  Bus Selector3/27 -> R_HALOUT_APS_CSOP_ApsSetData/27  "<VOUTP_DriIntend_enum>"
  Bus Selector3/53 -> Data Type Conversion35/1  "<VOUTP_TailgateSW_flg>"
  Data Type Conversion6/1 -> R_HALOUT_APS_CSOP_ApsSetData/74
  Bus Selector3/40 -> Data Type Conversion25/1  "<VOUTP_LatAccelV_flg>"
  Data Type Conversion105/1 -> R_HALOUT_APS_CSOP_ApsSetData/61
  Data Type Conversion104/1 -> R_HALOUT_APS_CSOP_ApsSetData/62
  Data Type Conversion118/1 -> R_HALOUT_APS_CSOP_ApsSetData/76
  Bus Selector3/2 -> R_HALOUT_APS_CSOP_ApsSetData/2  "<VOUTP_BrkPedalPos_pct>"
  Bus Selector3/3 -> R_HALOUT_APS_CSOP_ApsSetData/3  "<VOUTP_ActAPSPosn_pct>"
  Data Type Conversion17/1 -> R_HALOUT_APS_CSOP_ApsSetData/24
  Bus Selector3/56 -> R_HALOUT_APS_CSOP_ApsSetData/56  "<VOUTP_AVMParkingmode_enum>"
  Bus Selector3/22 -> Data Type Conversion15/1  "<VOUTP_LRPulseCount_enum>"
  [BOUTP_outputs] -> Bus Selector3/1
  Bus Selector3/71 -> R_HALOUT_APS_CSOP_ApsSetData/71  "<VOUTP_RRPressIndi_enum>"
  Bus Selector3/54 -> R_HALOUT_APS_CSOP_ApsSetData/54  "<VOUTP_AVMparkingcancel_enum>"
  Bus Selector3/50 -> R_HALOUT_APS_CSOP_ApsSetData/50  "<VOUTP_EPBSta_enum>"
  Bus Selector3/43 -> Data Type Conversion28/1  "<VOUTP_BrkSwSta_flg>"
  Data Type Conversion25/1 -> R_HALOUT_APS_CSOP_ApsSetData/40
  Data Type Conversion98/1 -> R_HALOUT_APS_CSOP_ApsSetData/68
  Ground_11/1 -> Data Type Conversion118/1
  Bus Selector3/11 -> Data Type Conversion19/1  "<VOUTP_RRRawWhlSpeedV_flg>"
  Bus Selector3/12 -> R_HALOUT_APS_CSOP_ApsSetData/12  "<VOUTP_LFWhlRotDir_enum>"
  Ground_16/1 -> Data Type Conversion122/1
  Bus Selector3/32 -> Data Type Conversion22/1  "<VOUTP_SASCAL_flg>"
  Bus Selector3/60 -> R_HALOUT_APS_CSOP_ApsSetData/60  "<VOUTP_IVIScreen_enum>"
  Data Type Conversion122/1 -> R_HALOUT_APS_CSOP_ApsSetData/81
  Bus Selector3/58 -> Data Type Conversion37/1  "<VOUTP_IVIStatus_flg>"
  Ground_14/1 -> Data Type Conversion121/1
  Data Type Conversion99/1 -> R_HALOUT_APS_CSOP_ApsSetData/67
  Ground6/1 -> Data Type Conversion96/1
  Data Type Conversion36/1 -> R_HALOUT_APS_CSOP_ApsSetData/57
  Bus Selector3/8 -> Data Type Conversion7/1  "<VOUTP_LFRawWhlSpeedV_flg>"
  Bus Selector3/33 -> Data Type Conversion23/1  "<VOUTP_SASV_flg>"
  Data Type Conversion27/1 -> R_HALOUT_APS_CSOP_ApsSetData/42
  Data Type Conversion18/1 -> R_HALOUT_APS_CSOP_ApsSetData/25
  Bus Selector3/9 -> Data Type Conversion8/1  "<VOUTP_RFRawWhlSpeedV_flg>"
  Bus Selector3/7 -> R_HALOUT_APS_CSOP_ApsSetData/7  "<VOUTP_RRRawWhlSpeed_kph>"
  Ground7/1 -> Data Type Conversion105/1
  Bus Selector3/6 -> R_HALOUT_APS_CSOP_ApsSetData/6  "<VOUTP_LRRawWhlSpeed_kph>"
  Ground8/1 -> Data Type Conversion17/1
  Bus Selector3/82 -> Terminator14/1  "<VOUTP_VehSpeed_kph>"
  Bus Selector3/63 -> Data Type Conversion103/1  "<VOUTP_TCSActive_flg>"
  Data Type Conversion8/1 -> R_HALOUT_APS_CSOP_ApsSetData/9
  Bus Selector3/41 -> Data Type Conversion26/1  "<VOUTP_LongAccelV_flg>"
  Data Type Conversion102/1 -> R_HALOUT_APS_CSOP_ApsSetData/64
  Bus Selector3/44 -> Data Type Conversion29/1  "<VOUTP_BrkSwV_flg>"
  Data Type Conversion31/1 -> R_HALOUT_APS_CSOP_ApsSetData/47
  Data Type Conversion22/1 -> R_HALOUT_APS_CSOP_ApsSetData/32
  Bus Selector3/72 -> R_HALOUT_APS_CSOP_ApsSetData/72  "<VOUTP_LRPressIndi_enum>"
  Bus Selector3/69 -> R_HALOUT_APS_CSOP_ApsSetData/69  "<VOUTP_RFPressIndi_enum>"
  Bus Selector3/48 -> Data Type Conversion32/1  "<VOUTP_EPBExtApplyAvail_flg>"
  Data Type Conversion10/1 -> R_HALOUT_APS_CSOP_ApsSetData/16
  Bus Selector3/37 -> R_HALOUT_APS_CSOP_ApsSetData/37  "<VOUTP_LongAccel_Gps>"
  Bus Selector3/30 -> R_HALOUT_APS_CSOP_ApsSetData/30  "<VOUTP_SASSpeed_degps>"
  Bus Selector3/46 -> R_HALOUT_APS_CSOP_ApsSetData/46  "<VOUTP_ESCAPSSta_enum>"
  Ground_17/1 -> Data Type Conversion124/1
  Bus Selector3/26 -> R_HALOUT_APS_CSOP_ApsSetData/26  "<VOUTP_ShifterHandleCmd_enum>"
  Bus Selector3/24 -> Terminator8/1  "<VOUTP_VehSpeed_kph>"
  Bus Selector3/14 -> R_HALOUT_APS_CSOP_ApsSetData/14  "<VOUTP_LRWhlRotDir_enum>"
  Data Type Conversion34/1 -> R_HALOUT_APS_CSOP_ApsSetData/52
  Bus Selector3/18 -> Data Type Conversion12/1  "<VOUTP_LRPulseCountV_flg>"
  Data Type Conversion33/1 -> R_HALOUT_APS_CSOP_ApsSetData/51
  Data Type Conversion13/1 -> R_HALOUT_APS_CSOP_ApsSetData/19
  Bus Selector3/51 -> Data Type Conversion33/1  "<VOUTP_AllDoorSW_flg>"
  Ground_13/1 -> Data Type Conversion120/1
  Bus Selector3/55 -> R_HALOUT_APS_CSOP_ApsSetData/55  "<VOUTP_AVMparkingexcute_enum>"
  Data Type Conversion28/1 -> R_HALOUT_APS_CSOP_ApsSetData/43
  Data Type Conversion32/1 -> R_HALOUT_APS_CSOP_ApsSetData/48
  Bus Selector3/28 -> R_HALOUT_APS_CSOP_ApsSetData/28  "<VOUTP_EPSAOIControl_enum>"
  Data Type Conversion29/1 -> R_HALOUT_APS_CSOP_ApsSetData/44
  Data Type Conversion103/1 -> R_HALOUT_APS_CSOP_ApsSetData/63
  Bus Selector3/1 -> R_HALOUT_APS_CSOP_ApsSetData/1  "<VOUTP_PowerSta_enum>"
  Bus Selector3/21 -> Data Type Conversion14/1  "<VOUTP_RFPulseCount_enum>"
  Bus Selector3/20 -> Data Type Conversion20/1  "<VOUTP_LFPulseCount_enum>"
  Bus Selector3/64 -> Data Type Conversion102/1  "<VOUTP_DriverSeatBeltCmd_flg>"
  Data Type Conversion14/1 -> R_HALOUT_APS_CSOP_ApsSetData/21
  Bus Selector3/65 -> Data Type Conversion101/1  "<VOUTP_DrDoorSW_flg>"
  Data Type Conversion23/1 -> R_HALOUT_APS_CSOP_ApsSetData/33
  Data Type Conversion35/1 -> R_HALOUT_APS_CSOP_ApsSetData/53
  Bus Selector3/77 -> Terminator10/1  "<VOUTP_VehSpeed_kph>"
  Bus Selector3/81 -> Terminator13/1  "<VOUTP_VehSpeed_kph>"
  Bus Selector3/83 -> Data Type Conversion117/1  "<VOUTP_IVIUserTakeOverAPSSta_flg>"
  Data Type Conversion96/1 -> R_HALOUT_APS_CSOP_ApsSetData/75
  Data Type Conversion124/1 -> R_HALOUT_APS_CSOP_ApsSetData/82
  Data Type Conversion101/1 -> R_HALOUT_APS_CSOP_ApsSetData/65
  Bus Selector3/5 -> R_HALOUT_APS_CSOP_ApsSetData/5  "<VOUTP_RFRawWhlSpeed_kph>"
  Data Type Conversion12/1 -> R_HALOUT_APS_CSOP_ApsSetData/18
  Bus Selector3/13 -> R_HALOUT_APS_CSOP_ApsSetData/13  "<VOUTP_RFWhlRotDir_enum>"
  Bus Selector3/66 -> Data Type Conversion100/1  "<VOUTP_PsDoorSW_flg>"
  Bus Selector3/19 -> Data Type Conversion13/1  "<VOUTP_RRPulseCountV_flg>"
  Bus Selector3/16 -> Data Type Conversion10/1  "<VOUTP_LFPulseCountV_flg>"
  Data Type Conversion19/1 -> R_HALOUT_APS_CSOP_ApsSetData/11
  Bus Selector3/67 -> Data Type Conversion99/1  "<VOUTP_RLDoorSW_flg>"
  Data Type Conversion24/1 -> R_HALOUT_APS_CSOP_ApsSetData/39
  Data Type Conversion26/1 -> R_HALOUT_APS_CSOP_ApsSetData/41
  Bus Selector3/70 -> R_HALOUT_APS_CSOP_ApsSetData/70  "<VOUTP_LFPressIndi_enum>"
  Bus Selector3/34 -> R_HALOUT_APS_CSOP_ApsSetData/34  "<VOUTP_GRADE_Deg>"
  Bus Selector3/68 -> Data Type Conversion98/1  "<VOUTP_RRDoorSW_flg>"
  Bus Selector3/52 -> Data Type Conversion34/1  "<VOUTP_HoodSW_flg>"
  Data Type Conversion37/1 -> R_HALOUT_APS_CSOP_ApsSetData/58
  Bus Selector3/39 -> Data Type Conversion24/1  "<VOUTP_YawRateV_flg>"
  Bus Selector3/62 -> Data Type Conversion104/1  "<VOUTP_ABSActive_flg>"
  Bus Selector3/49 -> R_HALOUT_APS_CSOP_ApsSetData/49  "<VOUTP_EPBErrSta_enum>"
  Bus Selector3/61 -> Terminator7/1  "<VOUTP_VehSpeedTimeOut_flg>"
  Bus Selector3/45 -> Data Type Conversion30/1  "<VOUTP_ESCStandstill_flg>"
  Bus Selector3/59 -> R_HALOUT_APS_CSOP_ApsSetData/59  "<VOUTP_CAASSw_enum>"
  Data Type Conversion120/1 -> R_HALOUT_APS_CSOP_ApsSetData/78
  Data Type Conversion9/1 -> R_HALOUT_APS_CSOP_ApsSetData/10
  Bus Selector3/36 -> R_HALOUT_APS_CSOP_ApsSetData/36  "<VOUTP_LatAccel_Gps>"
  Bus Selector3/15 -> R_HALOUT_APS_CSOP_ApsSetData/15  "<VOUTP_RRWhlRotDir_enum>"
  Data Type Conversion7/1 -> R_HALOUT_APS_CSOP_ApsSetData/8
  Data Type Conversion121/1 -> R_HALOUT_APS_CSOP_ApsSetData/79
  Data Type Conversion11/1 -> R_HALOUT_APS_CSOP_ApsSetData/17
  Bus Selector4/19 -> Data Type Conversion52/1  "<VOUTP_RFPulseCountTimeOut_flg>"
  Ground_23/1 -> Data Type Conversion116/1
  Data Type Conversion66/1 -> R_HALOUT_APS_CSOP_ApsSetTimeout/32
  Data Type Conversion91/1 -> R_HALOUT_APS_CSOP_ApsSetTimeout/43
  Data Type Conversion65/1 -> R_HALOUT_APS_CSOP_ApsSetTimeout/28
  Data Type Conversion53/1 -> R_HALOUT_APS_CSOP_ApsSetTimeout/20
  Ground_21/1 -> Data Type Conversion111/1
  Data Type Conversion74/1 -> R_HALOUT_APS_CSOP_ApsSetTimeout/41
  Bus Selector4/9 -> Data Type Conversion42/1  "<VOUTP_RRRawWhlSpeedVTimeOut_flg>"
  Bus Selector4/17 -> Data Type Conversion50/1  "<VOUTP_RRPulseCountVTimeOut_flg>"
  Bus Selector4/61 -> Terminator5/1  "<VOUTP_sigAmbAirT_C>"
  Data Type Conversion79/1 -> R_HALOUT_APS_CSOP_ApsSetTimeout/45
  Bus Selector4/6 -> Data Type Conversion40/1  "<VOUTP_LFRawWhlSpeedVTimeOut_flg>"
  Ground_18/1 -> Data Type Conversion109/1
  Bus Selector4/8 -> Data Type Conversion45/1  "<VOUTP_LRRawWhlSpeedVTimeOut_flg>"
  Data Type Conversion95/1 -> R_HALOUT_APS_CSOP_ApsSetTimeout/58
  Bus Selector4/13 -> Data Type Conversion56/1  "<VOUTP_RRWhlRotDirTimeOut_flg>"
  Data Type Conversion83/1 -> R_HALOUT_APS_CSOP_ApsSetTimeout/47
  Data Type Conversion42/1 -> R_HALOUT_APS_CSOP_ApsSetTimeout/9
  Data Type Conversion64/1 -> R_HALOUT_APS_CSOP_ApsSetTimeout/31
  Data Type Conversion80/1 -> R_HALOUT_APS_CSOP_ApsSetTimeout/46
  Bus Selector4/39 -> Data Type Conversion72/1  "<VOUTP_BrkSwStaTimeOut_flg>"
  Bus Selector4/21 -> Data Type Conversion54/1  "<VOUTP_RRPulseCountTimeOut_flg>"
  Data Type Conversion86/1 -> R_HALOUT_APS_CSOP_ApsSetTimeout/49
  Bus Selector4/18 -> Data Type Conversion55/1  "<VOUTP_LFPulseCountTimeOut_flg>"
  Bus Selector4/48 -> Data Type Conversion84/1  "<VOUTP_AVMparkingexcuteTimeOut_flg>"
  Data Type Conversion87/1 -> R_HALOUT_APS_CSOP_ApsSetTimeout/51
  Data Type Conversion43/1 -> R_HALOUT_APS_CSOP_ApsSetTimeout/10
  Data Type Conversion75/1 -> R_HALOUT_APS_CSOP_ApsSetTimeout/38
  Data Type Conversion90/1 -> R_HALOUT_APS_CSOP_ApsSetTimeout/56
  Bus Selector4/36 -> Data Type Conversion69/1  "<VOUTP_LatAccelVTimeOut_flg>"
  Data Type Conversion81/1 -> R_HALOUT_APS_CSOP_ApsSetTimeout/1
  Data Type Conversion56/1 -> R_HALOUT_APS_CSOP_ApsSetTimeout/13
  Bus Selector4/42 -> Data Type Conversion77/1  "<VOUTP_ESCAPSStaTimeOut_flg>"
  Data Type Conversion47/1 -> R_HALOUT_APS_CSOP_ApsSetTimeout/14
  Bus Selector4/12 -> Data Type Conversion46/1  "<VOUTP_LRWhlRotDirTimeOut_flg>"
  Bus Selector4/33 -> Data Type Conversion76/1  "<VOUTP_LongAccelTimeOut_flg>"
  Data Type Conversion116/1 -> R_HALOUT_APS_CSOP_ApsSetTimeout/67
  Bus Selector4/24 -> Data Type Conversion58/1  "<VOUTP_EPSAOIControlTimeOut_flg>"
  Bus Selector4/58 -> Terminator2/1  "<VOUTP_LFPressIndi_enum>"
  Ground4/1 -> Data Type Conversion95/1
  Data Type Conversion78/1 -> R_HALOUT_APS_CSOP_ApsSetTimeout/44
  Ground2/1 -> Data Type Conversion93/1
  Bus Selector4/52 -> Data Type Conversion88/1  "<VOUTP_CAASSwTimeOut_flg>"
  Data Type Conversion72/1 -> R_HALOUT_APS_CSOP_ApsSetTimeout/39
  Bus Selector4/35 -> Data Type Conversion68/1  "<VOUTP_YawRateVTimeOut_flg>"
  Data Type Conversion60/1 -> R_HALOUT_APS_CSOP_ApsSetTimeout/26
  Data Type Conversion109/1 -> R_HALOUT_APS_CSOP_ApsSetTimeout/62
  Bus Selector4/40 -> Data Type Conversion73/1  "<VOUTP_BrkSwVTimeOut_flg>"
  Data Type Conversion111/1 -> R_HALOUT_APS_CSOP_ApsSetTimeout/65
  Bus Selector4/38 -> Data Type Conversion75/1  "<VOUTP_MCPressureVTimeOut_flg>"
  Bus Selector4/27 -> Data Type Conversion61/1  "<VOUTP_SASSpeedValidTimeOut_flg>"
  Bus Selector4/55 -> Data Type Conversion85/1  "<VOUTP_TCSActiveTimeOut_flg>"
  Data Type Conversion41/1 -> R_HALOUT_APS_CSOP_ApsSetTimeout/7
  Data Type Conversion62/1 -> R_HALOUT_APS_CSOP_ApsSetTimeout/29
  Data Type Conversion71/1 -> R_HALOUT_APS_CSOP_ApsSetTimeout/23
  Data Type Conversion115/1 -> R_HALOUT_APS_CSOP_ApsSetTimeout/68
  Bus Selector4/49 -> Data Type Conversion86/1  "<VOUTP_AVMParkingmodeTimeOut_flg>"
  Bus Selector4/30 -> Data Type Conversion63/1  "<VOUTP_GRADETimeOut_flg>"
  Data Type Conversion70/1 -> R_HALOUT_APS_CSOP_ApsSetTimeout/37
  Data Type Conversion54/1 -> R_HALOUT_APS_CSOP_ApsSetTimeout/21
  Data Type Conversion68/1 -> R_HALOUT_APS_CSOP_ApsSetTimeout/35
  Ground5/1 -> Data Type Conversion106/1
  Bus Selector4/16 -> Data Type Conversion49/1  "<VOUTP_LRPulseCountVTimeOut_flg>"
  Bus Selector4/4 -> Data Type Conversion38/1  "<VOUTP_LRRawWhlSpeedTimeOut_flg>"
  Data Type Conversion51/1 -> R_HALOUT_APS_CSOP_ApsSetTimeout/3
  Data Type Conversion69/1 -> R_HALOUT_APS_CSOP_ApsSetTimeout/36
  Bus Selector4/29 -> Data Type Conversion62/1  "<VOUTP_SASVTimeOut_flg>"
  Bus Selector4/50 -> Data Type Conversion97/1  "<VOUTP_AVMErrSTATimeOut_flg>"
  Data Type Conversion82/1 -> R_HALOUT_APS_CSOP_ApsSetTimeout/54
  Bus Selector4/28 -> Data Type Conversion65/1  "<VOUTP_SASCALTimeOut_flg>"
  Bus Selector4/3 -> Data Type Conversion51/1  "<VOUTP_RFRawWhlSpeedTimeOut_flg>"
  Data Type Conversion40/1 -> R_HALOUT_APS_CSOP_ApsSetTimeout/6
  Data Type Conversion63/1 -> R_HALOUT_APS_CSOP_ApsSetTimeout/30
  [BOUTP_outputs] -> Bus Selector4/1
  Bus Selector4/1 -> Data Type Conversion81/1  "<VOUTP_BrkPedalPosTimeOut_flg>"
  Bus Selector4/10 -> Data Type Conversion43/1  "<VOUTP_LFWhlRotDirTimeOut_flg>"
  Data Type Conversion88/1 -> R_HALOUT_APS_CSOP_ApsSetTimeout/52
  Ground_20/1 -> Data Type Conversion112/1
  Bus Selector4/31 -> Data Type Conversion64/1  "<VOUTP_YawRateTimeOut_flg>"
  Data Type Conversion44/1 -> R_HALOUT_APS_CSOP_ApsSetTimeout/11
  Data Type Conversion113/1 -> R_HALOUT_APS_CSOP_ApsSetTimeout/63
  Data Type Conversion110/1 -> R_HALOUT_APS_CSOP_ApsSetTimeout/66
  Data Type Conversion48/1 -> R_HALOUT_APS_CSOP_ApsSetTimeout/15
  Bus Selector4/45 -> Data Type Conversion79/1  "<VOUTP_EPBErrStaTimeOut_flg>"
  Bus Selector4/34 -> Data Type Conversion67/1  "<VOUTP_MCPressureTimeOut_flg>"
  Ground_24/1 -> Data Type Conversion115/1
  Bus Selector4/56 -> Data Type Conversion90/1  "<VOUTP_DriverSeatBeltCmdTimeOut_flg>"
  Data Type Conversion93/1 -> R_HALOUT_APS_CSOP_ApsSetTimeout/60
  Data Type Conversion55/1 -> R_HALOUT_APS_CSOP_ApsSetTimeout/18
  Data Type Conversion73/1 -> R_HALOUT_APS_CSOP_ApsSetTimeout/40
  Bus Selector4/2 -> Data Type Conversion123/1  "<VOUTP_LFRawWhlSpeedTimeOut_flg>"
  Data Type Conversion57/1 -> R_HALOUT_APS_CSOP_ApsSetTimeout/22
  Bus Selector4/26 -> Data Type Conversion60/1  "<VOUTP_SASSpeedTimeOut_flg>"
  Bus Selector4/37 -> Data Type Conversion70/1  "<VOUTP_LongAccelVTimeOut_flg>"
  Bus Selector4/47 -> Data Type Conversion83/1  "<VOUTP_AVMparkingcancelTimeOut_flg>"
  Data Type Conversion61/1 -> R_HALOUT_APS_CSOP_ApsSetTimeout/27
  Data Type Conversion94/1 -> R_HALOUT_APS_CSOP_ApsSetTimeout/59
  Ground_26/1 -> Data Type Conversion114/1
  Data Type Conversion58/1 -> R_HALOUT_APS_CSOP_ApsSetTimeout/24
  Data Type Conversion123/1 -> R_HALOUT_APS_CSOP_ApsSetTimeout/2
  Bus Selector4/23 -> Data Type Conversion71/1  "<VOUTP_DriIntendTimeOut_flg>"
  Bus Selector4/46 -> Data Type Conversion80/1  "<VOUTP_EPBStaTimeOut_flg>"
  Ground_22/1 -> Data Type Conversion110/1
  Data Type Conversion106/1 -> R_HALOUT_APS_CSOP_ApsSetTimeout/57
  Bus Selector4/11 -> Data Type Conversion44/1  "<VOUTP_RFWhlRotDirTimeOut_flg>"
  Bus Selector4/20 -> Data Type Conversion53/1  "<VOUTP_LRPulseCountTimeOut_flg>"
  Bus Selector4/32 -> Data Type Conversion66/1  "<VOUTP_LatAccelTimeOut_flg>"
  Data Type Conversion46/1 -> R_HALOUT_APS_CSOP_ApsSetTimeout/12
  Bus Selector4/59 -> Terminator3/1  "<VOUTP_RRPressIndi_enum>"
  Bus Selector4/57 -> Terminator1/1  "<VOUTP_RFPressIndi_enum>"
  Bus Selector4/43 -> Data Type Conversion91/1  "<VOUTP_EPBExtReleaseAvailTimeOut_flg>"
  Bus Selector4/7 -> Data Type Conversion41/1  "<VOUTP_RFRawWhlSpeedVTimeOut_flg>"
  Bus Selector4/22 -> Data Type Conversion57/1  "<VOUTP_ShifterHandleCmdTimeOut_flg>"
  Bus Selector4/14 -> Data Type Conversion47/1  "<VOUTP_LFPulseCountVTimeOut_flg>"
  Data Type Conversion50/1 -> R_HALOUT_APS_CSOP_ApsSetTimeout/17
  Ground3/1 -> Data Type Conversion94/1
  Data Type Conversion38/1 -> R_HALOUT_APS_CSOP_ApsSetTimeout/4
  Data Type Conversion112/1 -> R_HALOUT_APS_CSOP_ApsSetTimeout/64
  Data Type Conversion84/1 -> R_HALOUT_APS_CSOP_ApsSetTimeout/48
  Data Type Conversion52/1 -> R_HALOUT_APS_CSOP_ApsSetTimeout/19
  Data Type Conversion97/1 -> R_HALOUT_APS_CSOP_ApsSetTimeout/50
  Data Type Conversion59/1 -> R_HALOUT_APS_CSOP_ApsSetTimeout/25
  Bus Selector4/51 -> Data Type Conversion87/1  "<VOUTP_IVIStatusTimeOut_flg>"
  Data Type Conversion49/1 -> R_HALOUT_APS_CSOP_ApsSetTimeout/16
  Ground_19/1 -> Data Type Conversion113/1
  Bus Selector4/15 -> Data Type Conversion48/1  "<VOUTP_RFPulseCountVTimeOut_flg>"
  Data Type Conversion92/1 -> R_HALOUT_APS_CSOP_ApsSetTimeout/61
  Data Type Conversion39/1 -> R_HALOUT_APS_CSOP_ApsSetTimeout/5
  Data Type Conversion114/1 -> R_HALOUT_APS_CSOP_ApsSetTimeout/69
  Bus Selector4/60 -> Terminator4/1  "<VOUTP_LRPressIndi_enum>"
  Data Type Conversion85/1 -> R_HALOUT_APS_CSOP_ApsSetTimeout/55
  Bus Selector4/44 -> Data Type Conversion78/1  "<VOUTP_EPBExtApplyAvailTimeOut_flg>"
  Data Type Conversion89/1 -> R_HALOUT_APS_CSOP_ApsSetTimeout/53
  Data Type Conversion77/1 -> R_HALOUT_APS_CSOP_ApsSetTimeout/42
  Bus Selector4/41 -> Data Type Conversion74/1  "<VOUTP_ESCStandstillTimeOut_flg>"
  Bus Selector4/5 -> Data Type Conversion39/1  "<VOUTP_RRRawWhlSpeedTimeOut_flg>"
  Bus Selector4/25 -> Data Type Conversion59/1  "<VOUTP_SASAngleTimeOut_flg>"
  Data Type Conversion45/1 -> R_HALOUT_APS_CSOP_ApsSetTimeout/8
  Bus Selector4/53 -> Data Type Conversion89/1  "<VOUTP_IVIScreenTimeOut_flg>"
  Bus Selector4/54 -> Data Type Conversion82/1  "<VOUTP_ABSActiveTimeOut_flg>"
  Data Type Conversion76/1 -> R_HALOUT_APS_CSOP_ApsSetTimeout/33
  Ground1/1 -> Data Type Conversion92/1
  Data Type Conversion67/1 -> R_HALOUT_APS_CSOP_ApsSetTimeout/34
  From139/1 -> Bus Selector8/1
  Detect Increase1/1 -> R_HALOUTCDD_CSOP_ResetPedalZeroPosDone/Enable
  Bus Selector8/1 -> Detect Increase1/1  "<VOUTP_ResetPedalZeroPosStart_flg>"
  Unit Delay4/1 -> R_DIDWriteCDD_CSOP_DIDSet_NVMPedalZP/Enable
  Bus Selector9/1 -> R_DIDWriteCDD_CSOP_DIDSet_NVMPedalZP/1(In3)  "<VHAL_DIDSetNVMPedalZP_raw8>"
  [u8_ReadPedalZeroPosReq] -> Data Type Conversion108/1
  Data Type Conversion108/1 -> Unit Delay4/1
  [BOUTP_DIDSetData_outputs] -> Bus Selector9/1
  Bus Selector6/1 -> Data Type Conversion107/1  "<VHAL_TPMSSensorIDRegResults_raw8>"
  [BOUTP_DIDSetData_outputs] -> Bus Selector6/1
  Data Type Conversion107/1 -> R_HALOUTCDD_CSOP_TPMSSensorIDRegSetResults/1(In1)
  R_UDSCDD_CSOP_SetDTCStatus/1(Out1) -> Terminator_16/1
  Ground10/1 -> R_HALOUTCDD_CSOP_SleepRequest/1(SleepState)
  OUTP_AFTER/12(DTC_Constant_Array) -> [DTC_Constant_Array]
  [DTC_Constant_Array] -> R_UDSCDD_CSOP_SetDTCStatus/3(DTC_Const)
  HAL_OUT/45 -> [E2E_CAN3_VCU1_Trigger]
  HAL_OUT/46 -> [E2E_CAN3_VCU1_toNIDEC_Trigger]
  HAL_OUT/47 -> [E2E_CAN4_VCU1_Trigger]
  HAL_OUT/44 -> IRV_E2E_CAN4_SG_FD4_CE100_0_write/1
  HAL_OUT/43 -> IRV_E2E_CAN3_SG_FD3_VCU1_toNIDEC_write/1
  HAL_OUT/42 -> IRV_E2E_CAN3_SG_FD3_VCU1_write/1
  HAL_OUT/41 -> IRV_ms5000_CAN2_SG_FD2_Version_write/1
  HAL_OUT/40 -> IRV_ms500_CAN1_SG_FD1_VMC2_write/1
  HAL_OUT/39 -> IRV_ms20_CAN2_SG_FD2_C20_0_write/1
  HAL_OUT/38 -> IRV_ms20_CAN1_SG_FD1_APS2_write/1
  HAL_OUT/37 -> IRV_ms1000_CAN3_SG_GW_IVI6_toNIDEC_write/1
  HAL_OUT/36 -> IRV_ms100_CAN5_SG_GW5_CE100_0_write/1
  HAL_OUT/35 -> IRV_ms100_CAN3_SG_FD3_THCM1_write/1
  HAL_OUT/34 -> IRV_ms100_CAN2_SG_GW2_CE100_1_write/1

== system SWC_HALOUT_type_backup/run_SWC_HALOUT_UDS_10ms_sys ==
  function : TriggerPort  TriggerType=function-call  VariantControl=(inherit)  SampleTimeType=periodic  SampleTime=-1
  R_HALINCDD_CSOP_UDS_Main : FunctionCaller  FunctionPrototype=R_HALINCDD_CSOP_UDS_Main()

== system SWC_HALOUT_type_backup/P_WDGCDD/run_SWC_HALOUT_AppCallWDG_End_sys ==
  function : TriggerPort  TriggerType=function-call  IsSimulinkFunction=on  FunctionName=run_SWC_HALOUT_AppCallWDG_End  VariantControl=(inherit)
